simulink library "lib_controller"  (R2015a)
settings: Solver=ode45  StartTime=0.0  StopTime=10.0  RelTol=1e-3
values from neighbouring files (symbols this model uses):
  CG_0 = [0,0,0.02]'    [SetupComplete.m]
  g = 9.81    [SetupComplete.m]
  h_M = 0.064    [SetupComplete.m]
  I_BAC_0 = [ Ix,0,Ixz;0,Iy,0;Ixz,0,Iz]    [SetupComplete.m]
  l = 0.3450    (= 0.345)    [NDI_components.m]    (also in SetupComplete.m; robust_controller.m)
  m = 3.51    [SetupComplete.m]
  m_0 = 2.61    [SetupComplete.m]
  m_M = 0.300    (= 0.3)    [SetupComplete.m]
  T_sim = 0.01    [Run3Copter.m]
undefined symbols (not defined in the file or in its folder): Theta_1_roll_last, Theta_2_roll_last, Theta_3_roll_last, V_long_lastA_w_z, V_long_lastAoA, V_roll_last, V_yaw_last, W_long_lastA_w_z, W_long_lastAoA, W_roll_last, W_yaw_last
libraries: simulink x65, Adaptive_FaultTolerantControl x8, lib_controller x5, qcatlib x4, dspinverses x4, aerolibtransform2 x3, aerolib6dofsys x1
(part 2 of 10)

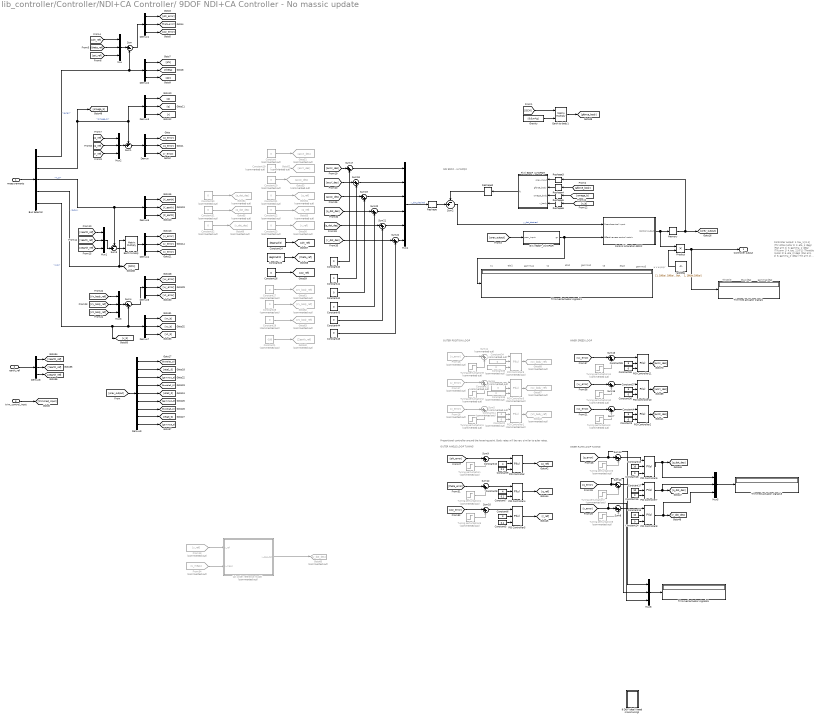
== system lib_controller/Controller/NDI+CA Controller/ 9DOF NDI+CA Controller - No massic update ==
  note: gamma3
  note: gamma2
  note: gamma1
  note: eta3
  note: eta2
  note: eta1
  note: t3
  note: t2
  note: t1
  note: u
      | v
      | w
      | p
      | q
      | r
  note: OUTER POSITION LOOP
  note: gamma[deg]
  note: eta [deg]
  note: Throttle
  note: Controller output:
      | 1. tau_1 [0-1] (Thr ottle motor 1)
      | 2. eta_1 (deg)  (Pan arm 1)
      | 3. gamma_1 (deg)  (Tilt arm 1)
      |
      | 4. tau_2 [0-1] (Throttle motor 2)
      | 5. eta_2 (deg)  (Pan arm 2)
      | 6. gamma_2 (deg)  (Tilt arm 2)
      |
      | 7. tau_3 [0-1] (Throttle motor 3)
      | 8. eta_3 (deg)  (Pan arm  3)
      | 9. gamma_3 (deg)  (Tilt arm 3)
  note: Proportional controller around the hovering point. Body rates will be very similar to euler rates.
  note: INNER RATE LOOP TUNING
  note: OUTER ANGLE LOOP TUNING
  note: INNER SPEED LOOP
  note: NDI 9DOF - UVWPQR
  measurements : Inport
  earth_ref : Inport  Port=2
  trim_control_input : Inport  Port=3
  1st order reference model : Subsystem  Commented=on  mask(1st order model reference block){Kref=1, Kb=20, fi=0.25, fc=0.5, Kf=1}
      mask prompts: Kref "1st order reference gain"; Kb "Bandwidth gain"; fi "Integral gain"; fc "Command FF gain"; Kf "Command_dot FF gain"
      mask help:
      | Generates a desired first order derivative of a commanded output taking
      | into account the current measured output.
      | Kref is the gain that determines the first order system between y_ref and
      | y_commanded signals. Ycom/Yref = Kref/(1 + Kref)
      | fi and fc can be defaulted to 0.25 and 0.5 for a critically damped 2nd
      | order response between y_meas and the error signal (y_com - y_meas) considering
      | a perfect dynamic inversion.
      mask Help:
      | Juan Herrero Macias <jn.herrerom@gmail.com>
      | This architecture can be found and explained in Fault-tolerant Flight
      | Control and Guidance Systems, Ducard, Guillaume.
      mask TypeOptions Kref: Kref gain/Gain
      mask TypeOptions Kb: Bandwidth gain/Gain
      mask TypeOptions fi: Integral gain/Gain
      mask TypeOptions fc: Command FF gain/Gain
      mask TypeOptions Kf: Command_dot FF gain/Gain
  9 DOF Ideal (Need more tuning) : Subsystem
  Bus Selector : BusSelector  OutputSignals=euler,omega_b,X_e,DCM,V_b
  Constant{,2,11..12,19..23,27..35} (18 alike) : Constant  Commented=on  Value=0
  Constant1 : Constant  Commented=on  Value=-100
  Constant10 : Constant  Value=4
  Constant13 : Constant  Value=10
  Constant{3,14,16,18,26,36,38,40..45} (13 alike) : Constant  Value=0
  Constant15 : Constant  Value=10
  Constant17 : Constant  Value=10
  Constant24 : Constant  Value=deg2rad(0)
  Constant25 : Constant  Value=deg2rad(0)
  Constant37 : Constant  Value=5
  Constant39 : Constant  Value=5
  Constant4 : Constant  Value=5
  Constant5 : Constant  Value=0.1
  Constant6 : Constant  Value=3
  Constant7 : Constant  Value=0.1
  Constant8 : Constant  Value=4
  Constant9 : Constant  Value=0.1
  Control Allocation 9DOF : Subsystem  Variant=on  OverrideUsingVariant=(default)
  Demux{,1..8} (9 alike) : Demux  Outputs=3
  Demux9 : Demux  Outputs=9
  Earth to body : Product  Multiplication=Matrix(*)
  Earth to body1 : Product  Multiplication=Matrix(*)
  F(X) 9DOF_UVWPQR : MATLAB Function  TreatAsAtomicUnit=on
  From13 : From  Commented=on  GotoTag=y_ref
  From16 : From  Commented=on  GotoTag=z_error
  From17 : From  Commented=on  GotoTag=y_error
  From18 : From  Commented=on  GotoTag=x_error
  From34 : From  Commented=on  GotoTag=y_meas
  G(X) 9DOF_UVWPQR : MATLAB Function  TreatAsAtomicUnit=on
  Goto40 : Goto  Commented=on  GotoTag=Zearth_ref
  Goto43 : Goto  Commented=on  GotoTag=Vz_body_ref
  Goto51 : Goto  Commented=on  GotoTag=accX_des
  Goto52 : Goto  Commented=on  GotoTag=accY_des
  Goto53 : Goto  Commented=on  GotoTag=accZ_des
  Goto54 : Goto  Commented=on  GotoTag=p_ref
  Goto55 : Goto  Commented=on  GotoTag=q_ref
  Goto56 : Goto  Commented=on  GotoTag=r_ref
  Goto60 : Goto  Commented=on  GotoTag=y_dot_des
  Goto61 : Goto  Commented=on  GotoTag=Vx_body_ref
  Goto62 : Goto  Commented=on  GotoTag=Vy_body_ref
  Goto63 : Goto  Commented=on  GotoTag=Vz_body_ref
  Goto64 : Goto  Commented=on  GotoTag=p_dot_des
  Goto65 : Goto  Commented=on  GotoTag=q_dot_des
  Goto66 : Goto  Commented=on  GotoTag=r_dot_des
  Goto67 : Goto  Commented=on  GotoTag=Vy_body_ref
  Goto68 : Goto  Commented=on  GotoTag=Vx_body_ref
  Gravity : Constant  Value=[0;0;m*g]
  Memory : Memory  X0=[0,0,0,0,0,0,0,0,0]  LinearizeAsDelay=on
  Mux{,1..3,5,8} (6 alike) : Mux  Inputs=3
  Mux4 : Mux  Inputs=6
  PID Controller{,2,4..8,10..11} (9 alike) : simulink/Continuous/PID Controller  Controller=PI  TimeDomain=Continuous-time  SampleTime=-1  IntegratorMethod=Forward Euler  FilterMethod=Forward Euler  Form=Parallel  UseFilter=on  ControllerParametersSource=external  P=1  I=1  D=0  N=100  InitialConditionSource=internal  InitialConditionForIntegrator=0  InitialConditionForFilter=0  ExternalReset=none  LimitOutput=off  UpperSaturationLimit=inf  LowerSaturationLimit=-inf  LinearizeAsGain=on  AntiWindupMode=none  Kb=1  TrackingMode=off  Kt=1  PParamMin=[]  PParamMax=[]  IParamMin=[]  IParamMax=[]  DParamMin=[]  DParamMax=[]  NParamMin=[]  NParamMax=[]  KbParamMin=[]  KbParamMax=[]  KtParamMin=[]  KtParamMax=[]  POutMin=[]  POutMax=[]  IOutMin=[]  IOutMax=[]  DOutMin=[]  DOutMax=[]  NOutMin=[]  NOutMax=[]  KbOutMin=[]  KbOutMax=[]  KtOutMin=[]  KtOutMax=[]  IntegratorOutMin=[]  IntegratorOutMax=[]  FilterOutMin=[]  FilterOutMax=[]  SumOutMin=[]  SumOutMax=[]  SumI1OutMin=[]  SumI1OutMax=[]  SumI2OutMin=[]  SumI2OutMax=[]  SumI3OutMin=[]  SumI3OutMax=[]  SumDOutMin=[]  SumDOutMax=[]  SaturationOutMin=[]  SaturationOutMax=[]  IntegratorContinuousStateAttributes=''  IntegratorStateMustResolveToSignalObject=off  IntegratorRTWStateStorageClass=Auto  FilterContinuousStateAttributes=''  FilterStateMustResolveToSignalObject=off  FilterRTWStateStorageClass=Auto  DifferentiatorICPrevScaledInput=0  DifferentiatorOutMin=[]  DifferentiatorOutMax=[]
  PID Controller1 : simulink/Continuous/PID Controller  Commented=on  Controller=PI  TimeDomain=Continuous-time  SampleTime=-1  IntegratorMethod=Forward Euler  FilterMethod=Forward Euler  Form=Parallel  UseFilter=on  ControllerParametersSource=external  P=1  I=1  D=0  N=100  InitialConditionSource=internal  InitialConditionForIntegrator=0  InitialConditionForFilter=0  ExternalReset=none  LimitOutput=off  UpperSaturationLimit=inf  LowerSaturationLimit=-inf  LinearizeAsGain=on  AntiWindupMode=none  Kb=1  TrackingMode=off  Kt=1  PParamMin=[]  PParamMax=[]  IParamMin=[]  IParamMax=[]  DParamMin=[]  DParamMax=[]  NParamMin=[]  NParamMax=[]  KbParamMin=[]  KbParamMax=[]  KtParamMin=[]  KtParamMax=[]  POutMin=[]  POutMax=[]  IOutMin=[]  IOutMax=[]  DOutMin=[]  DOutMax=[]  NOutMin=[]  NOutMax=[]  KbOutMin=[]  KbOutMax=[]  KtOutMin=[]  KtOutMax=[]  IntegratorOutMin=[]  IntegratorOutMax=[]  FilterOutMin=[]  FilterOutMax=[]  SumOutMin=[]  SumOutMax=[]  SumI1OutMin=[]  SumI1OutMax=[]  SumI2OutMin=[]  SumI2OutMax=[]  SumI3OutMin=[]  SumI3OutMax=[]  SumDOutMin=[]  SumDOutMax=[]  SaturationOutMin=[]  SaturationOutMax=[]  IntegratorContinuousStateAttributes=''  IntegratorStateMustResolveToSignalObject=off  IntegratorRTWStateStorageClass=Auto  FilterContinuousStateAttributes=''  FilterStateMustResolveToSignalObject=off  FilterRTWStateStorageClass=Auto  DifferentiatorICPrevScaledInput=0  DifferentiatorOutMin=[]  DifferentiatorOutMax=[]
  PID Controller3 : simulink/Continuous/PID Controller  Commented=on  Controller=PI  TimeDomain=Continuous-time  SampleTime=-1  IntegratorMethod=Forward Euler  FilterMethod=Forward Euler  Form=Parallel  UseFilter=on  ControllerParametersSource=external  P=1  I=1  D=0  N=100  InitialConditionSource=internal  InitialConditionForIntegrator=0  InitialConditionForFilter=0  ExternalReset=none  LimitOutput=off  UpperSaturationLimit=inf  LowerSaturationLimit=-inf  LinearizeAsGain=on  AntiWindupMode=none  Kb=1  TrackingMode=off  Kt=1  PParamMin=[]  PParamMax=[]  IParamMin=[]  IParamMax=[]  DParamMin=[]  DParamMax=[]  NParamMin=[]  NParamMax=[]  KbParamMin=[]  KbParamMax=[]  KtParamMin=[]  KtParamMax=[]  POutMin=[]  POutMax=[]  IOutMin=[]  IOutMax=[]  DOutMin=[]  DOutMax=[]  NOutMin=[]  NOutMax=[]  KbOutMin=[]  KbOutMax=[]  KtOutMin=[]  KtOutMax=[]  IntegratorOutMin=[]  IntegratorOutMax=[]  FilterOutMin=[]  FilterOutMax=[]  SumOutMin=[]  SumOutMax=[]  SumI1OutMin=[]  SumI1OutMax=[]  SumI2OutMin=[]  SumI2OutMax=[]  SumI3OutMin=[]  SumI3OutMax=[]  SumDOutMin=[]  SumDOutMax=[]  SaturationOutMin=[]  SaturationOutMax=[]  IntegratorContinuousStateAttributes=''  IntegratorStateMustResolveToSignalObject=off  IntegratorRTWStateStorageClass=Auto  FilterContinuousStateAttributes=''  FilterStateMustResolveToSignalObject=off  FilterRTWStateStorageClass=Auto  DifferentiatorICPrevScaledInput=0  DifferentiatorOutMin=[]  DifferentiatorOutMax=[]
  PID Controller9 : simulink/Continuous/PID Controller  Commented=on  Controller=PI  TimeDomain=Continuous-time  SampleTime=-1  IntegratorMethod=Forward Euler  FilterMethod=Forward Euler  Form=Parallel  UseFilter=on  ControllerParametersSource=external  P=1  I=1  D=0  N=100  InitialConditionSource=internal  InitialConditionForIntegrator=0  InitialConditionForFilter=0  ExternalReset=none  LimitOutput=off  UpperSaturationLimit=inf  LowerSaturationLimit=-inf  LinearizeAsGain=on  AntiWindupMode=none  Kb=1  TrackingMode=off  Kt=1  PParamMin=[]  PParamMax=[]  IParamMin=[]  IParamMax=[]  DParamMin=[]  DParamMax=[]  NParamMin=[]  NParamMax=[]  KbParamMin=[]  KbParamMax=[]  KtParamMin=[]  KtParamMax=[]  POutMin=[]  POutMax=[]  IOutMin=[]  IOutMax=[]  DOutMin=[]  DOutMax=[]  NOutMin=[]  NOutMax=[]  KbOutMin=[]  KbOutMax=[]  KtOutMin=[]  KtOutMax=[]  IntegratorOutMin=[]  IntegratorOutMax=[]  FilterOutMin=[]  FilterOutMax=[]  SumOutMin=[]  SumOutMax=[]  SumI1OutMin=[]  SumI1OutMax=[]  SumI2OutMin=[]  SumI2OutMax=[]  SumI3OutMin=[]  SumI3OutMax=[]  SumDOutMin=[]  SumDOutMax=[]  SaturationOutMin=[]  SaturationOutMax=[]  IntegratorContinuousStateAttributes=''  IntegratorStateMustResolveToSignalObject=off  IntegratorRTWStateStorageClass=Auto  FilterContinuousStateAttributes=''  FilterStateMustResolveToSignalObject=off  FilterRTWStateStorageClass=Auto  DifferentiatorICPrevScaledInput=0  DifferentiatorOutMin=[]  DifferentiatorOutMax=[]
  Product : Product
  Reshape : Reshape  OutputDimensionality=Column vector (2-D)
  Reshape2 : Reshape  OutputDimensionality=Column vector (2-D)  OutputDimensions=[6,1]
  Reshape{3..6} (4 alike) : Reshape  OutputDimensions=[6,1]
  Sum : Sum  Inputs=|+-
  Sum1 : Sum  Inputs=-+|
  Sum{7..10,12..22} (15 alike) : Sum  Inputs=|++
  Sum11 : Sum  Commented=on  Inputs=|++
  Sum2 : Sum  Inputs=-+|
  Sum3 : Sum  Inputs=-+|
  Sum4 : Sum  Inputs=|+-
  Sum5 : Sum  Commented=on  Inputs=|++
  Sum6 : Sum  Commented=on  Inputs=|++
  Trimmed actuator signals{,1,3,5} (4 alike) : Display
  Tuning perturbation{,5..6,8} (4 alike) : Step  Commented=on  Time=20  After=3*pi/180  SampleTime=0
  Tuning perturbation{1..3,9..11} (6 alike) : Step  Commented=on  Time=20  SampleTime=0
  Tuning perturbation4 : Step  Commented=on  Time=20  After=-3*pi/180  SampleTime=0
  Tuning perturbation7 : Step  Commented=on  Time=20  After=-3*pi/180  SampleTime=0
  rad2deg : Constant  Value="[1, 180/pi, 180/pi,    1,180/pi, 180/pi,     1, 180/pi,180/pi]"
  Controller output : Outport
  wires:
  PID Controller9/1 -> Goto68/1
  Tuning perturbation9/1 -> Sum11/2
  From18/1 -> Sum11/1
  Sum11/1 -> PID Controller9/1
  Constant35/1 -> PID Controller9/3
  Constant34/1 -> PID Controller9/2
  PID Controller3/1 -> Goto67/1
  Tuning perturbation2/1 -> Sum6/2
  From17/1 -> Sum6/1
  Sum6/1 -> PID Controller3/1
  Constant33/1 -> PID Controller3/3
  Constant12/1 -> PID Controller3/2
  PID Controller1/1 -> Goto43/1
  Tuning perturbation1/1 -> Sum5/2
  Sum5/1 -> PID Controller1/1
  Constant2/1 -> PID Controller1/3
  Constant11/1 -> PID Controller1/2
  Constant1/1 -> Goto40/1
  G(X) 9DOF_UVWPQR/1(gx) -> Trimmed actuator signals1/1, Control Allocation 9DOF/2(Effectiveness control matrix)
  [prev_output] -> G(X) 9DOF_UVWPQR/1(prev_input)
  Control Allocation 9DOF/1(Control output) -> Memory/1, Product/1
  Sum2/1 -> Control Allocation 9DOF/1(Pseudocontrol input)  "y_dot_desired"
  Constant13/1 -> PID Controller6/2
  Sum3/1 -> Earth to body/2
  Constant32/1 -> Goto66/1
  Constant31/1 -> Goto65/1
  Constant30/1 -> Goto64/1
  Memory/1 -> [prev_output], Reshape3/1
  [DCM] -> Earth to body1/1
  Mux8/1 -> Trimmed actuator signals5/1
  [r_error] -> Sum8/1, Mux8/3
  [q_error] -> Sum13/1, Mux8/2
  [p_error] -> Sum14/1, Mux8/1
  [psi_error] -> Sum10/1
  [theta_error] -> Sum12/1
  [phi_error] -> Sum9/1
  Constant29/1 -> Goto63/1
  Constant28/1 -> Goto62/1
  Constant27/1 -> Goto61/1
  PID Controller2/1 -> [accZ_des]
  Mux5/1 -> Trimmed actuator signals3/1
  1st order reference model/1(y_des_dot) -> Goto60/1
  From34/1 -> 1st order reference model/2(y_meas)
  From13/1 -> 1st order reference model/1(y_ref)
  rad2deg/1 -> Product/2
  Product/1 -> Controller output/1, Trimmed actuator signals/1
  Constant18/1 -> PID Controller6/3
  Constant26/1 -> [psi_ref]
  Constant25/1 -> [theta_ref]
  Constant24/1 -> [phi_ref]
  Constant23/1 -> Goto56/1
  Constant22/1 -> Goto55/1
  Constant21/1 -> Goto54/1
  Constant20/1 -> Goto53/1
  Constant19/1 -> Goto52/1
  Constant/1 -> Goto51/1
  [v_b] -> Reshape6/1
  Reshape6/1 -> F(X) 9DOF_UVWPQR/4(v_body)
  Reshape5/1 -> F(X) 9DOF_UVWPQR/3(omega_body)
  Reshape4/1 -> F(X) 9DOF_UVWPQR/2(gforce_body)
  [omega_b] -> Reshape5/1
  Reshape3/1 -> F(X) 9DOF_UVWPQR/1(prev_input)
  Reshape2/1 -> Sum2/1
  Reshape/1 -> Sum2/2
  Mux4/1 -> Reshape/1  "y_dot_desired"
  Tuning perturbation7/1 -> Sum13/2
  Tuning perturbation6/1 -> Sum14/2
  Tuning perturbation8/1 -> Sum8/2
  Sum13/1 -> PID Controller7/1
  Sum8/1 -> PID Controller8/1
  Sum14/1 -> PID Controller6/1
  Constant16/1 -> PID Controller7/3
  Constant17/1 -> PID Controller7/2
  Constant14/1 -> PID Controller8/3
  Constant15/1 -> PID Controller8/2
  PID Controller8/1 -> [r_dot_des], Mux5/3
  PID Controller7/1 -> [q_dot_des], Mux5/2
  PID Controller6/1 -> [p_dot_des], Mux5/1
  Tuning perturbation4/1 -> Sum12/2
  Tuning perturbation/1 -> Sum9/2
  Tuning perturbation5/1 -> Sum10/2
  Sum12/1 -> PID Controller4/1
  Sum10/1 -> PID Controller5/1
  Sum9/1 -> PID Controller/1
  Constant7/1 -> PID Controller4/3
  Constant9/1 -> PID Controller/3
  Constant10/1 -> PID Controller/2
  Constant8/1 -> PID Controller4/2
  Constant5/1 -> PID Controller5/3
  Constant6/1 -> PID Controller5/2
  PID Controller5/1 -> [r_ref]
  PID Controller4/1 -> [q_ref]
  PID Controller/1 -> [p_ref]
  Tuning perturbation3/1 -> Sum7/2
  [vz_error] -> Sum7/1
  Sum7/1 -> PID Controller2/1
  Constant3/1 -> PID Controller2/3
  Constant4/1 -> PID Controller2/2
  [gforce_body] -> Reshape4/1
  Earth to body1/1 -> [gforce_body]
  Gravity/1 -> Earth to body1/2
  F(X) 9DOF_UVWPQR/1(fx) -> Reshape2/1
  Mux/1 -> Sum/1
  Demux3/3 -> [r]
  Demux3/2 -> [q]
  Demux3/1 -> [p]
  Demux2/1 -> [phi]
  Demux2/2 -> [theta]
  Demux2/3 -> [psi]
  measurements/1 -> Bus Selector/1
  Bus Selector/1 -> Demux2/1, Sum/2  "<euler>"
  Bus Selector/2 -> Demux3/1, Sum1/1, [omega_b]  "<omega_b>"
  Sum1/1 -> Demux/1
  Sum/1 -> Demux1/1
  Demux/3 -> [r_error]
  Demux/2 -> [q_error]
  Demux/1 -> [p_error]
  Demux1/1 -> [phi_error]
  Demux1/2 -> [theta_error]
  Demux1/3 -> [psi_error]
  trim_control_input/1 -> [trimmed_input]
  [theta_ref] -> Mux/2
  [phi_ref] -> Mux/1
  [psi_ref] -> Mux/3
  Mux2/1 -> Sum1/2
  [q_ref] -> Mux2/2
  [p_ref] -> Mux2/1
  [r_ref] -> Mux2/3
  Bus Selector/3 -> Demux5/1, Sum3/1  "<X_e>"
  Demux5/3 -> [Z_earth]
  Demux5/2 -> [Y_earth]
  Demux5/1 -> [X_earth]
  Demux4/3 -> [z_error]
  Demux4/2 -> [y_error]
  Demux4/1 -> [x_error]
  Mux1/1 -> Sum3/2
  [Yearth_ref] -> Mux1/2
  [Xearth_ref] -> Mux1/1
  [Zearth_ref] -> Mux1/3
  Mux3/1 -> Sum4/1
  Demux7/1 -> [vx_b]
  Demux7/2 -> [vy_b]
  Demux7/3 -> [vz_b]
  Bus Selector/5 -> Demux7/1, Sum4/2, [v_b]  "<V_b>"
  Sum4/1 -> Demux6/1
  Demux6/1 -> [vx_error]
  Demux6/2 -> [vy_error]
  Demux6/3 -> [vz_error]
  [Vy_body_ref] -> Mux3/2
  [Vx_body_ref] -> Mux3/1
  [Vz_body_ref] -> Mux3/3
  Bus Selector/4 -> [DCM], Earth to body/1  "<DCM>"
  Earth to body/1 -> Demux4/1
  Demux8/3 -> [Zearth_ref]
  Demux8/2 -> [Yearth_ref]
  Demux8/1 -> [Xearth_ref]
  earth_ref/1 -> Demux8/1
  [prev_output] -> Demux9/1
  Demux9/1 -> [throttle1_0]
  Demux9/2 -> [eta1_0]
  Demux9/3 -> [gamma1_0]
  Demux9/4 -> [throttle2_0]
  Demux9/5 -> [eta2_0]
  Demux9/6 -> [gamma2_0]
  Demux9/7 -> [throttle3_0]
  Demux9/8 -> [eta3_0]
  Demux9/9 -> [gamma3_0]
  PID Controller10/1 -> [accY_des]
  Tuning perturbation10/1 -> Sum15/2
  [vy_error] -> Sum15/1
  Sum15/1 -> PID Controller10/1
  Constant36/1 -> PID Controller10/3
  Constant37/1 -> PID Controller10/2
  PID Controller11/1 -> [accX_des]
  Tuning perturbation11/1 -> Sum16/2
  [vx_error] -> Sum16/1
  Sum16/1 -> PID Controller11/1
  Constant38/1 -> PID Controller11/3
  Constant39/1 -> PID Controller11/2
  From16/1 -> Sum5/1
  [accX_des] -> Sum17/1
  [accY_des] -> Sum18/1
  [accZ_des] -> Sum19/1
  [p_dot_des] -> Sum20/1
  [q_dot_des] -> Sum21/1
  [r_dot_des] -> Sum22/1
  Constant40/1 -> Sum17/2
  Constant41/1 -> Sum18/2
  Constant42/1 -> Sum19/2
  Constant43/1 -> Sum20/2
  Constant44/1 -> Sum21/2
  Constant45/1 -> Sum22/2
  Sum22/1 -> Mux4/6
  Sum21/1 -> Mux4/5
  Sum20/1 -> Mux4/4
  Sum19/1 -> Mux4/3
  Sum18/1 -> Mux4/2
  Sum17/1 -> Mux4/1

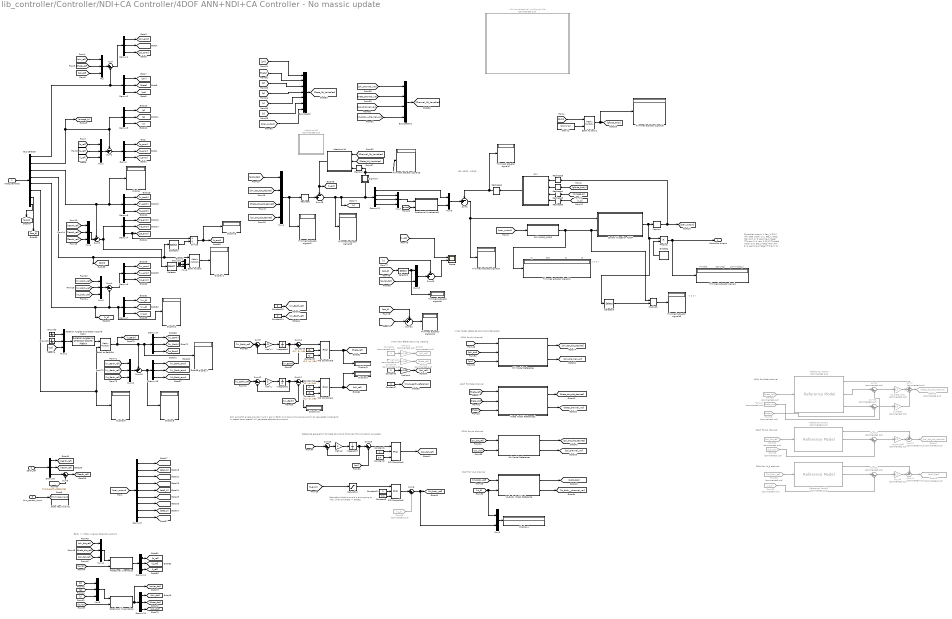
== system lib_controller/Controller/NDI+CA Controller/4DOF ANN+NDI+CA Controller - No massic update ==
  note: Roll and pitch angle provide X and Y acc in Earth axis (around hovering point). So requested increments in speed (error speed) will generate attitude commands
  note: Saturation block to avoid z_error going to
      |  infty when phi/theta -> 90deg
  note: Inner loop reference tuning / testing
  note: Earth <-> Body Angular Rate Conversions
  note: Reference generation for Rate Command Channels (for simulation purposes)
  note: ACAH for phi channel
  note: NDI 4DOF - WPQR
  note: Controller output:
      | 1. tau_1 [0-1] (Thr ottle motor 1)
      | 2. eta_1 (deg)  (Pan arm 1)
      | 3. gamma_1 (deg)  (Tilt arm 1)
      |
      | 4. tau_2 [0-1] (Throttle motor 2)
      | 5. eta_2 (deg)  (Pan arm 2)
      | 6. gamma_2 (deg)  (Tilt arm 2)
      |
      | 7. tau_3 [0-1] (Throttle motor 3)
      | 8. eta_3 (deg)  (Pan arm  3)
      | 9. gamma_3 (deg)  (Tilt arm 3)
  note: Throttle
  note: eta [deg]
  note: gamma[deg]
  note: eta1
  note: t3
  note: t2
  note: t1
  note: w
      | p
      | q
      | r
  note: ACAH for theta channel
  note: RCAH for psi channel
  note: RCAH for Vz_b channel
  note: Inner Model reference Command Generator
  note: ACAH for theta channel
  note: RCAH for psi channel
  note: RCAH for Vz_b channel
  note: w
      | p
      | q
      | r
  measurements : Inport
  earth_ref : Inport  Port=2
  trim_control_input : Inport  Port=3
  Adaptive NN : Subsystem  Variant=on  VariantControl=Variant  OverrideUsingVariant=NN on AoA
      mask Display:
      | image(imread('ANN.png'))
      | 
      | 
      | port_label('input', 2, 'State vars')
      | port_label('input', 1, 'Channel vars')
      | port_label('input', 3, 'v prev')
      | 
      | port_label('output', 1, 'v_ad^')
  Adaptive NN1 : Subsystem  Commented=on  Variant=on  VariantControl=Variant  OverrideUsingVariant=NN on AoA
      mask Display:
      | image(imread('ANN.png'))
      | 
      | 
      | port_label('input', 2, 'State vars')
      | port_label('input', 1, 'Channel vars')
      | port_label('input', 3, 'v prev')
      | 
      | port_label('output', 1, 'v_ad^')
  Bus Creator : BusCreator  Inputs=7
  Bus Creator1 : BusCreator
  Bus Selector : BusSelector  OutputSignals=euler,omega_b,X_e,DCM,V_b,V_e,A_b,A_s
  Constant1 : Constant  Value=4
  Constant10 : Constant  Value=10 * pi /180
  Constant11 : Constant
  Constant12 : Constant  Value=0.2 * pi /180
  Constant13 : Constant  Value=5
  Constant14 : Constant  Value=0
  Constant2 : Constant  Value=0.4
  Constant3 : Constant  Value=0.1
  Constant4 : Constant  Commented=on  Value=0
  Constant5 : Constant  Commented=on  Value=0
  Constant6 : Constant  Value=0
  Constant7 : Constant  Value=0
  Constant8 : Constant  Value=-10 * pi /180
  Constant9 : Constant  Value=-0.2 * pi /180
  Control Allocation 4DOF : Subsystem  Variant=on  OverrideUsingVariant=Variant1
  Demux{,1..8,10..11,13..14} (13 alike) : Demux  Outputs=3
  Demux12 : Demux
  Demux9 : Demux  Outputs=9
  Display{,1..10} (11 alike) : Display
  Divide : Product  Inputs=*/
  Earth to EarthPsi : Product  Multiplication=Matrix(*)
  Earth to body : Product  Multiplication=Matrix(*)
  Earth to body1 : Product  Multiplication=Matrix(*)
  F(X) : MATLAB Function  TreatAsAtomicUnit=on
  From29 : From  Commented=on  GotoTag=theta
  From33 : From  Commented=on  GotoTag=psi_dot_ref
  From36 : From  Commented=on  GotoTag=Vz_body_ref
  From38 : From  Commented=on  GotoTag=theta_ref
  From39 : From  Commented=on  GotoTag=vz_b
  From47 : From  Commented=on  GotoTag=theta_dot
  From49 : From  Commented=on  GotoTag=psi_dot
  From65 : From  Commented=on  GotoTag=vz_b
  G(X) 4DOF_WPQR : MATLAB Function  TreatAsAtomicUnit=on
  Goto Tag Visibility : GotoTagVisibility  GotoTag=trimmed_input
  Goto45 : Goto  Commented=on  GotoTag=theta_dot_dot_desired
  Goto47 : Goto  Commented=on  GotoTag=psi_dot_dot_desired
  Goto48 : Goto  Commented=on  GotoTag=accZ_des
  Goto57 : Goto  Commented=on  GotoTag=phi_ref
  Goto58 : Goto  Commented=on  GotoTag=theta_ref
  Gravity : Constant  Value=[0;0;m*g]
  Ground{,1..3} (4 alike) : Ground
  Integrator1 : Integrator
  Integrator2 : Integrator
  Integrator7 : Integrator
  Ki_theta1 : Gain  Commented=on  Gain=0.5
  Kp_psi_dot1 : Gain  Commented=on  Gain=0.5
  Kp_theta_dot1 : Gain  Commented=on  Gain=0.5
  Kp_vz1 : Gain  Commented=on  Gain=0.5
  Kref psi : Gain
  Kref psi1 : Gain  Commented=on  Gain=pi/180
  Kref psi2 : Gain  Commented=on  Gain=pi/180
  Kref psi4 : Gain  Gain=pi/180
  Kref vx : Gain  Gain=-5
  Kref vy : Gain  Gain=5
  Memory : Memory  X0=[0,0,0,0,0,0,0,0,0]  LinearizeAsDelay=on
  Memory1 : Memory
  Mux{,1..3,5..7,10..12} (10 alike) : Mux  Inputs=3
  Mux13 : Mux  Inputs=2
  Mux4 : Mux
  Mux8 : Mux  Inputs=2
  Mux9 : Mux  Inputs=2
  On-line (adaptive) multi-layer NNs : Subsystem  Commented=on
      mask Display:
      | image(imread('ANN.png'))
      | 
      | port_label('input', 1, 'v prev')
      | port_label('input', 2, 'All meas')
      | port_label('input', 3, 'NN vars')
      | 
      | port_label('output', 1, 'v_ad^')
  PID Controller{1..4} (4 alike) : simulink/Continuous/PID Controller  Controller=PI  TimeDomain=Continuous-time  SampleTime=-1  IntegratorMethod=Forward Euler  FilterMethod=Forward Euler  Form=Parallel  UseFilter=on  ControllerParametersSource=external  P=1  I=1  D=0  N=100  InitialConditionSource=internal  InitialConditionForIntegrator=0  InitialConditionForFilter=0  ExternalReset=none  LimitOutput=off  UpperSaturationLimit=inf  LowerSaturationLimit=-inf  LinearizeAsGain=on  AntiWindupMode=none  Kb=1  TrackingMode=off  Kt=1  PParamMin=[]  PParamMax=[]  IParamMin=[]  IParamMax=[]  DParamMin=[]  DParamMax=[]  NParamMin=[]  NParamMax=[]  KbParamMin=[]  KbParamMax=[]  KtParamMin=[]  KtParamMax=[]  POutMin=[]  POutMax=[]  IOutMin=[]  IOutMax=[]  DOutMin=[]  DOutMax=[]  NOutMin=[]  NOutMax=[]  KbOutMin=[]  KbOutMax=[]  KtOutMin=[]  KtOutMax=[]  IntegratorOutMin=[]  IntegratorOutMax=[]  FilterOutMin=[]  FilterOutMax=[]  SumOutMin=[]  SumOutMax=[]  SumI1OutMin=[]  SumI1OutMax=[]  SumI2OutMin=[]  SumI2OutMax=[]  SumI3OutMin=[]  SumI3OutMax=[]  SumDOutMin=[]  SumDOutMax=[]  SaturationOutMin=[]  SaturationOutMax=[]  IntegratorContinuousStateAttributes=''  IntegratorStateMustResolveToSignalObject=off  IntegratorRTWStateStorageClass=Auto  FilterContinuousStateAttributes=''  FilterStateMustResolveToSignalObject=off  FilterRTWStateStorageClass=Auto  DifferentiatorICPrevScaledInput=0  DifferentiatorOutMin=[]  DifferentiatorOutMax=[]
  Phi Model Reference : Subsystem  mask{omega_n=8, xi=1.1, r=1}
      mask prompts: omega_n "Natural Frequency"; xi "Damping"; r "NN Error dynamic ratio"
      mask help:
      | 2nd Order Model Reference System
      | Natural frequency and damping ratio set the dynamic of the model reference.
      | Error dynamic ratio sets how faster compared to the reference model dynamics
      | is the settling time of the inversion error provided by the NN.
      mask Display:
      | TF = tf([omega_n^2],[1 xi*omega_n omega_n^2]);
      | 
      | [y,t]=step(TF);
      | S = stepinfo(y,t);
      | 
      | pos = get_param(gcb, 'Position');
      | width = pos(3) - pos(1);
      | height = pos(4) - pos(2);
      | t = t.*width/max(t);
      | y=y.*height/max(y);
      | plot(t,y);
      | S2 = stepinfo(y,t);
      | 
      | if S.Overshoot==0 % 1st order response
      |     text(S2.RiseTime ,height*0.85,['Rise time = ',num2str(S.RiseTime),'s' ]);
      |     text(S2.RiseTime ,height*0.75,['Settling Time = ',num2str(S.SettlingTime)]);
      | 
      | elseif S.Overshoot<0.05 % 2nd order response
      |     text(width*0.5 ,height*0.9,['Rise time = ',num2str(S.RiseTime),'s' ]);
      |     text(width*0.5 ,height*0.8,['Pike time = ',num2str(S.PeakTime),'s' ]);
      |     text(width*0.5 ,height*0.7,['Os = ',num2str(S.Peak)]);
      |     text(width*0.5 ,height*0.6,['SettlingTime = ',num2str(S.SettlingTime)]);
      | else % 2nd order response
      |     text(S2.PeakTime ,S2.Peak*0.85,['Peak time = ',num2str(S.PeakTime),'s' ]);
      |     text(S2.PeakTime ,S2.Peak*0.75,['Os = ',num2str(S.Peak)]);
      |     text(S2.PeakTime ,S2.Peak*0.65,['SettlingTime = ',num2str(S.SettlingTime)]);
      | end
      | 
      | 
      | [num,den] = tfdata(TF);
      | dpoly(num{:},den{:}, 's');
  Product : Product
  Product1 : Product  Multiplication=Matrix(*)
  Psi Model Reference : Subsystem  mask{tau=0.15, r=1}
      mask prompts: tau "Time Constant"; r "NN Error dynamic ratio"
      mask help:
      | 1st Order Model Reference System
      | Tau is the time constant and sets the dynamics of the reference model.
      | Error dynamic ratio sets how faster compared to the reference model is the
      | NN output going to try to compensate for the inversion error.
      mask Display:
      | K_ref=1/tau;
      | TF = tf([K_ref],[1 K_ref]);
      | 
      | [y,t]=step(TF);
      | S = stepinfo(y,t);
      | 
      | pos = get_param(gcb, 'Position');
      | width = pos(3) - pos(1);
      | height = pos(4) - pos(2);
      | t = t.*width/max(t);
      | y=y.*height/max(y);
      | plot(t,y);
      | S2 = stepinfo(y,t);
      | 
      | if S.Overshoot==0 % 1st order response
      |     text(S2.RiseTime ,height*0.85,['Rise time = ',num2str(S.RiseTime),'s' ]);
      |     text(S2.RiseTime ,height*0.75,['Settling Time = ',num2str(S.SettlingTime)]);
      | 
      | elseif S.Overshoot<0.05 % 2nd order response
      |     text(width*0.5 ,height*0.9,['Rise time = ',num2str(S.RiseTime),'s' ]);
      |     text(width*0.5 ,height*0.8,['Pike time = ',num2str(S.PeakTime),'s' ]);
      |     text(width*0.5 ,height*0.7,['Os = ',num2str(S.Peak)]);
      |     text(width*0.5 ,height*0.6,['SettlingTime = ',num2str(S.SettlingTime)]);
      | else % 2nd order response
      |     text(S2.PeakTime ,S2.Peak*0.85,['Peak time = ',num2str(S.PeakTime),'s' ]);
      |     text(S2.PeakTime ,S2.Peak*0.75,['Os = ',num2str(S.Peak)]);
      |     text(S2.PeakTime ,S2.Peak*0.65,['SettlingTime = ',num2str(S.SettlingTime)]);
      | end
      | 
      | 
      | [num,den] = tfdata(TF);
      | dpoly(num{:},den{:}, 's');
  Reference Model1 : Adaptive_FaultTolerantControl/Ref Model and P Controller/Reference Model  Commented=on  omega_n=omega_n  xi=xi
  Reference Model4 : Adaptive_FaultTolerantControl/Ref Model and P Controller/Reference Model  Commented=on  omega_n=2.5  xi=1.1
  Reference Model5 : Adaptive_FaultTolerantControl/Ref Model and P Controller/Reference Model  Commented=on  omega_n=omega_n  xi=xi
  Reshape : Reshape
  Reshape2 : Reshape  OutputDimensionality=Column vector (2-D)  OutputDimensions=[6,1]
  Reshape{3..6} (4 alike) : Reshape  OutputDimensions=[6,1]
  Rotation Angles to Direction Cosine Matrix : aerolibtransform2/Rotation Angles to Direction Cosine Matrix  rotationOrder=ZYX
  Rotational Kinematics : MATLAB Function  TreatAsAtomicUnit=on
  Rotational Kinematics1 : MATLAB Function  TreatAsAtomicUnit=on
  Rotational Kinematics2 : MATLAB Function  TreatAsAtomicUnit=on
  Saturation : Saturate  UpperLimit=4  LowerLimit=-4
  Scope : Scope  NumInputPorts=2
      settings: ShowLegends=on  YMin=-5~-20  YMax=15~20  SaveName=ScopeData5
  Selector : Selector  InputPortWidth=3  Indices=[3]
  Selector1 : Selector  NumberOfDimensions=2  InputPortWidth=[9]  IndexOptions=Index vector (dialog),Index vector (dialog)  Indices=3,3  OutputSizes=1,1
  Selector2 : Selector  InputPortWidth=3  Indices=[3]
  Selector3 : Selector  InputPortWidth=9  Indices=[1 2 4 7]
  "Sigmoid " : Subsystem  mask{a=0.15}
      mask prompts: a "Sigmoid a param"
      mask TypeOptions a: a/Value
      mask Display:
      | x=-25:0.1:25;
      | 
      | y=(2.0 ./ (1.0 + exp(-a.*x))-1) ;
      | y2=zeros(size(x));
      | 
      | plot(x,y,x,y2);
      | 
      | %text(-20,0.5, ['a= ',num2str(a)])
  Sum{,4..5,10,12,17,25..26} (8 alike) : Sum  Inputs=|+-
  Sum{1..3,18..20} (6 alike) : Sum  Inputs=-+|
  Sum11 : Sum  Commented=on  Inputs=+-|
  Sum{8,13,15..16} (4 alike) : Sum  Commented=on  Inputs=|+-
  Sum14 : Sum  Commented=on  Inputs=+-|
  Sum21 : Sum  Inputs=++|
  Sum6 : Sum  Inputs=|++
  Sum7 : Sum  Commented=on  Inputs=+--
  Sum9 : Sum  Inputs=|++
  Theta Model Reference1 : Subsystem  mask{omega_n=8, xi=1.1, r=1}
      mask prompts: omega_n "Natural Frequency"; xi "Damping"; r "NN Error dynamic ratio"
      mask help:
      | 2nd Order Model Reference System
      | Natural frequency and damping ratio set the dynamic of the model reference.
      | Error dynamic ratio sets how faster compared to the reference model dynamics
      | is the settling time of the inversion error provided by the NN.
      mask Display:
      | TF = tf([omega_n^2],[1 xi*omega_n omega_n^2]);
      | 
      | [y,t]=step(TF);
      | S = stepinfo(y,t);
      | 
      | pos = get_param(gcb, 'Position');
      | width = pos(3) - pos(1);
      | height = pos(4) - pos(2);
      | t = t.*width/max(t);
      | y=y.*height/max(y);
      | plot(t,y);
      | S2 = stepinfo(y,t);
      | 
      | if S.Overshoot==0 % 1st order response
      |     text(S2.RiseTime ,height*0.85,['Rise time = ',num2str(S.RiseTime),'s' ]);
      |     text(S2.RiseTime ,height*0.75,['Settling Time = ',num2str(S.SettlingTime)]);
      | 
      | elseif S.Overshoot<0.05 % 2nd order response
      |     text(width*0.5 ,height*0.9,['Rise time = ',num2str(S.RiseTime),'s' ]);
      |     text(width*0.5 ,height*0.8,['Pike time = ',num2str(S.PeakTime),'s' ]);
      |     text(width*0.5 ,height*0.7,['Os = ',num2str(S.Peak)]);
      |     text(width*0.5 ,height*0.6,['SettlingTime = ',num2str(S.SettlingTime)]);
      | else % 2nd order response
      |     text(S2.PeakTime ,S2.Peak*0.85,['Peak time = ',num2str(S.PeakTime),'s' ]);
      |     text(S2.PeakTime ,S2.Peak*0.75,['Os = ',num2str(S.Peak)]);
      |     text(S2.PeakTime ,S2.Peak*0.65,['SettlingTime = ',num2str(S.SettlingTime)]);
      | end
      | 
      | 
      | [num,den] = tfdata(TF);
      | dpoly(num{:},den{:}, 's');
  Trimmed actuator signals{,1..10} (11 alike) : Display
  Vz_body Model Reference : Subsystem  mask{tau=0.3, r=1}
      mask prompts: tau "Time Constant"; r "NN Error dynamic ratio"
      mask help:
      | 1st Order Model Reference System
      | Tau is the time constant and sets the dynamics of the reference model.
      | Error dynamic ratio sets how faster compared to the reference model is the
      | NN output going to try to compensate for the inversion error.
      mask Display:
      | K_ref=1/tau;
      | TF = tf([K_ref],[1 K_ref]);
      | 
      | [y,t]=step(TF);
      | S = stepinfo(y,t);
      | 
      | pos = get_param(gcb, 'Position');
      | width = pos(3) - pos(1);
      | height = pos(4) - pos(2);
      | t = t.*width/max(t);
      | y=y.*height/max(y);
      | plot(t,y);
      | S2 = stepinfo(y,t);
      | 
      | if S.Overshoot==0 % 1st order response
      |     text(S2.RiseTime ,height*0.85,['Rise time = ',num2str(S.RiseTime),'s' ]);
      |     text(S2.RiseTime ,height*0.75,['Settling Time = ',num2str(S.SettlingTime)]);
      | 
      | elseif S.Overshoot<0.05 % 2nd order response
      |     text(width*0.5 ,height*0.9,['Rise time = ',num2str(S.RiseTime),'s' ]);
      |     text(width*0.5 ,height*0.8,['Pike time = ',num2str(S.PeakTime),'s' ]);
      |     text(width*0.5 ,height*0.7,['Os = ',num2str(S.Peak)]);
      |     text(width*0.5 ,height*0.6,['SettlingTime = ',num2str(S.SettlingTime)]);
      | else % 2nd order response
      |     text(S2.PeakTime ,S2.Peak*0.85,['Peak time = ',num2str(S.PeakTime),'s' ]);
      |     text(S2.PeakTime ,S2.Peak*0.75,['Os = ',num2str(S.Peak)]);
      |     text(S2.PeakTime ,S2.Peak*0.65,['SettlingTime = ',num2str(S.SettlingTime)]);
      | end
      | 
      | 
      | [num,den] = tfdata(TF);
      | dpoly(num{:},den{:}, 's');
  rad2deg : Constant  Value=[1, 180/pi, 0,1,0, 0, 1, 0,0]
  Controller output : Outport
  tag scope: trimmed_input=scoped
  wires:
  Demux9/9 -> [gamma3_0]
  Demux9/8 -> [eta3_0]
  Demux9/7 -> [throttle3_0]
  Demux9/6 -> [gamma2_0]
  Demux9/5 -> [eta2_0]
  Demux9/4 -> [throttle2_0]
  Demux9/3 -> [gamma1_0]
  Demux9/2 -> [eta1_0]
  Demux9/1 -> [throttle1_0]
  [prev_output] -> Demux9/1
  earth_ref/1 -> Demux8/1
  Demux8/1 -> [Xearth_ref]
  Demux8/2 -> [Yearth_ref]
  Bus Selector/4 -> Earth to body/1, Selector1/1, [DCM]  "<DCM>"
  [Vz_body_ref] -> Mux3/3
  [Vx_body_ref] -> Mux3/1
  [Vy_body_ref] -> Mux3/2
  Demux6/3 -> [vz_error]
  Demux6/2 -> [vy_error]
  Demux6/1 -> [vx_error]
  Sum4/1 -> Demux6/1
  Bus Selector/5 -> [v_b], Sum4/2, Display2/1, Demux7/1  "<V_b>"
  Demux7/3 -> [vz_b]
  Demux7/2 -> [vy_b]
  Demux7/1 -> [vx_b]
  Mux3/1 -> Sum4/1
  [Zearth_ref] -> Mux1/3
  [Xearth_ref] -> Mux1/1
  [Yearth_ref] -> Mux1/2
  Mux1/1 -> Sum3/2
  Demux4/1 -> [Xe_error]
  Demux4/2 -> [Ye_error]
  Demux4/3 -> Divide/1, [Ze_error]
  Demux5/1 -> [X_earth]
  Demux5/2 -> [Y_earth]
  Demux5/3 -> [Z_earth]
  Bus Selector/3 -> Display/1, Demux5/1, Sum3/1  "<X_e>"
  [r_ref] -> Mux2/3
  [p_ref] -> Mux2/1
  [q_ref] -> Mux2/2
  Mux2/1 -> Sum1/2
  [psi_ref] -> Mux/3
  [phi_ref] -> Mux/1
  [theta_ref] -> Mux/2
  trim_control_input/1 -> [trimmed_input]
  Demux1/3 -> [psi_error]
  Demux1/2 -> [theta_error]
  Demux1/1 -> [phi_error]
  Demux/1 -> [p_error]
  Demux/2 -> [q_error]
  Demux/3 -> [r_error]
  Sum/1 -> Demux1/1
  Sum1/1 -> Demux/1
  Bus Selector/2 -> [omega_b], Sum1/1, Demux3/1  "<omega_b>"
  Bus Selector/1 -> Sum/2, Demux2/1  "<euler>"
  measurements/1 -> Bus Selector/1
  Demux2/3 -> [psi]
  Demux2/2 -> [theta]
  Demux2/1 -> [phi]
  Demux3/1 -> [p]
  Demux3/2 -> [q]
  Demux3/3 -> [r]
  Mux/1 -> Sum/1
  F(X)/1(fx) -> Reshape2/1
  Gravity/1 -> Earth to body1/2
  Earth to body1/1 -> Trimmed actuator signals6/1, [gforce_body]
  [gforce_body] -> Reshape4/1
  Mux4/1 -> Trimmed actuator signals2/1, Reshape/1  "y_dot_desired"
  Reshape2/1 -> Sum2/1, Trimmed actuator signals7/1
  Reshape3/1 -> F(X)/1(prev_input)
  [omega_b] -> Reshape5/1
  Reshape4/1 -> F(X)/2(gforce_body)
  Reshape5/1 -> F(X)/3(omega_body)
  Reshape6/1 -> F(X)/4(v_body)
  [v_b] -> Reshape6/1
  Product/1 -> Trimmed actuator signals/1, Controller output/1
  rad2deg/1 -> Product/2
  [DCM] -> Earth to body1/1
  Memory/1 -> Reshape3/1, [prev_output]
  Sum3/1 -> Demux4/1, Selector/1
  Sum2/1 -> Trimmed actuator signals4/1, Control Allocation 4DOF/1(Pseudocontrol input)  "y_dot_desired"
  Control Allocation 4DOF/1(Control output) -> Selector3/1, Product/1, Memory/1
  [prev_output] -> G(X) 4DOF_WPQR/1(prev_input)
  [accZ_des] -> Mux4/1
  G(X) 4DOF_WPQR/1(gx) -> Trimmed actuator signals1/1, Product1/1, Control Allocation 4DOF/2(Effectiveness control matrix)
  Selector/1 -> Mux6/3
  Ground/1 -> Mux6/1
  Ground1/1 -> Mux6/2
  Mux6/1 -> Earth to body/2
  Earth to body/1 -> Display1/1
  Sum18/1 -> Trimmed actuator signals3/1, Demux12/1, "Sigmoid "/1(In), [v]  "upsilon"
  Reshape/1 -> Sum18/2  "v_o"
  Adaptive NN/1(v_ad^) -> [v_ad], Sum18/1  "v_ad"
  "Sigmoid "/1(Out) -> Trimmed actuator signals5/1, Memory1/1
  Memory1/1 -> Adaptive NN/3(v_ad^ prev)
  [euler] -> Rotational Kinematics/2(Euler)
  Demux11/1 -> [p_ref]
  Demux11/2 -> [q_ref]
  Demux11/3 -> [r_ref]
  Rotational Kinematics/1(PQR) -> Demux11/1
  [phi_dot_ref] -> Mux11/1
  [theta_dot_ref] -> Mux11/2
  [psi_dot_ref] -> Mux11/3
  Mux11/1 -> Rotational Kinematics/1(Eulerdot)
  [euler] -> Rotational Kinematics1/2(Euler)
  Mux5/1 -> Rotational Kinematics1/1(PQR)
  [r] -> Mux5/3
  [p] -> Mux5/1
  [q] -> Mux5/2
  Demux10/1 -> [phi_dot]
  Demux10/2 -> [theta_dot]
  Demux10/3 -> [psi_dot]
  Rotational Kinematics1/1(Eulerdot) -> [euler_dot], Demux10/1
  Theta Model Reference1/1(y_dot_dot_des) -> [theta_dot_dot_desired]
  [phi_dot_dot_desired] -> Mux4/2
  [theta_dot_dot_desired] -> Mux4/3
  [psi_dot_dot_desired] -> Mux4/4
  Demux12/2 -> Mux7/1  "v_phi"
  Demux12/3 -> Mux7/2  "v_theta"
  Demux12/4 -> Mux7/3  "v_psi"
  Mux7/1 -> Rotational Kinematics2/1(Eulerdot)
  [euler] -> Rotational Kinematics2/2(Euler)
  Mux8/1 -> Sum2/2  "upsilon_b"
  Demux12/1 -> Mux8/1  "v_z"
  Rotational Kinematics2/1(PQR) -> Mux8/2  "upsilon_body"
  Integrator7/1 -> Sum26/1, Sum25/2  "psi_c"
  Kref psi/1 -> Integrator7/1
  Sum25/1 -> Kref psi/1
  [psi_ref] -> Sum25/1
  [psi] -> Sum26/2
  PID Controller1/1 -> [psi_dot_ref]  "psi_dot_ref"
  Constant1/1 -> PID Controller1/2
  Constant2/1 -> PID Controller1/3
  Sum26/1 -> PID Controller1/1  "psi_error"
  Vz_body Model Reference/1(y_dot_des) -> [accZ_des]
  [Vz_body_ref] -> Vz_body Model Reference/1(u_ref)
  Constant11/1 -> PID Controller2/2
  Constant3/1 -> PID Controller2/3
  [z_error] -> Saturation/1
  PID Controller2/1 -> Sum6/1
  Selector1/1 -> Divide/2
  Divide/1 -> Display3/1, [z_error]
  [phi_ref] -> Phi Model Reference/1(u_ref)
  [phi_dot] -> Phi Model Reference/2(y_dot)
  [phi] -> Phi Model Reference/3(y)
  Phi Model Reference/1(y_dot_dot_des) -> [phi_dot_dot_desired]
  From29/1 -> Sum16/2
  Sum16/1 -> Ki_theta1/1  "theta_error"
  From38/1 -> Reference Model4/1
  Reference Model4/2 -> Sum8/1  "theta_dot_c"
  From47/1 -> Sum8/2
  Sum8/1 -> Kp_theta_dot1/1  "theta_dot_error"
  Ki_theta1/1 -> Sum7/3
  Kp_theta_dot1/1 -> Sum7/2
  Sum7/1 -> Goto45/1
  Reference Model1/2 -> Sum13/1  "psi_dot_c"
  Reference Model1/1 -> Sum11/1  "psi_dot_dot_c"
  From49/1 -> Sum13/2
  Sum13/1 -> Kp_psi_dot1/1  "psi_dot_error"
  Kp_psi_dot1/1 -> Sum11/2
  Sum11/1 -> Goto47/1
  Reference Model4/3 -> Sum16/1  "theta_c"
  From33/1 -> Reference Model1/1
  Reference Model5/2 -> Sum15/1  "vz_b_c"
  Reference Model5/1 -> Sum14/1  "accZ_c"
  From39/1 -> Sum15/2
  Sum15/1 -> Kp_vz1/1  "vz_error"
  Kp_vz1/1 -> Sum14/2
  Sum14/1 -> Goto48/1
  From36/1 -> Reference Model5/1
  Reference Model4/1 -> Sum7/1  "theta_dot_dot"
  [theta_ref] -> Theta Model Reference1/1(u_ref)
  [theta_dot] -> Theta Model Reference1/2(y_dot)
  [theta] -> Theta Model Reference1/3(y)
  [psi_dot_ref] -> Psi Model Reference/1(u_ref)
  [psi_dot] -> Psi Model Reference/2(y_dot)
  Psi Model Reference/1(y_dot_des) -> [psi_dot_dot_desired]
  [vz_b] -> Mux9/1, Vz_body Model Reference/2(y_dot)
  Phi Model Reference/2(NN_variables) -> [phi_channel_var]
  Vz_body Model Reference/2(NN_variables) -> [Vz_body__channel_var]
  Psi Model Reference/2(NN_variables) -> [psi_channel_var]
  Theta Model Reference1/2(NN_variables) -> [theta_channel_var]
  [p] -> Bus Creator/3  "p"
  [theta] -> Bus Creator/2  "theta"
  [q] -> Bus Creator/4  "q"
  [phi] -> Bus Creator/1  "phi"
  [r] -> Bus Creator/5  "r"
  Bus Creator/1 -> [State_NN_Variables]
  [State_NN_Variables] -> Adaptive NN/2(System State Vars)
  [Vz_body__channel_var] -> Bus Creator1/4  "vertical acc channel"
  [psi_channel_var] -> Bus Creator1/3  "yaw channel"
  [theta_channel_var] -> Bus Creator1/2  "pitch channel"
  [phi_channel_var] -> Bus Creator1/1  "roll channel"
  Bus Creator1/1 -> [Channel_NN_Variables]
  [Channel_NN_Variables] -> Adaptive NN/1(Model Reference Vars)
  [prev_output] -> Bus Creator/7  "prev_outputs"
  [w] -> Bus Creator/6  "w"
  Constant4/1 -> Kref psi1/1
  Constant5/1 -> Kref psi2/1
  Constant6/1 -> Kref psi4/1
  Kref psi1/1 -> Goto57/1
  Kref psi2/1 -> Goto58/1
  Kref psi4/1 -> [psi_ref]
  Mux9/1 -> Display4/1
  Demux8/3 -> Sum5/1
  Sum5/1 -> [Zearth_ref]
  Constant7/1 -> [Inc_Z_earth_reference]
  [Inc_Z_earth_reference] -> Sum5/2
  From65/1 -> Sum6/2
  Sum6/1 -> Mux9/2, [Vz_body_ref]
  Integrator1/1 -> Sum10/1, Sum9/2  "vx_c"
  Kref vx/1 -> Integrator1/1
  Sum9/1 -> Kref vx/1
  [Vx_Earth_ref] -> Sum9/1
  [Vx_Earth] -> Sum10/2
  Constant8/1 -> PID Controller3/2
  Constant9/1 -> PID Controller3/3
  Sum10/1 -> PID Controller3/1  "vx_error"
  Integrator2/1 -> Sum17/1, Sum12/2  "vy_c"
  Kref vy/1 -> Integrator2/1
  Sum12/1 -> Kref vy/1
  [Vy_Earth_ref] -> Sum12/1
  [Vy_Earth] -> Sum17/2
  Constant10/1 -> PID Controller4/2
  Constant12/1 -> PID Controller4/3
  Sum17/1 -> Display10/1, PID Controller4/1  "vy_error"
  Constant13/1 -> [Vx_Earth_ref]
  Constant14/1 -> [Vy_Earth_ref]
  Saturation/1 -> PID Controller2/1
  [Vz_Earth_ref] -> Mux10/3
  [Vx_Earth_ref] -> Mux10/1
  [Vy_Earth_ref] -> Mux10/2
  Demux13/3 -> [Vz_Earth_error]
  Demux13/2 -> [Vy_Earth_error]
  Demux13/1 -> [Vx_Earth_error]
  Sum19/1 -> Display6/1, Demux13/1
  Bus Selector/6 -> Earth to EarthPsi/2, Display5/1  "<V_e>"
  Demux14/3 -> [Vz_Earth]
  Demux14/2 -> [Vy_Earth]
  Demux14/1 -> [Vx_Earth]
  Ground3/1 -> Mux12/1
  Ground2/1 -> Mux12/2
  [psi] -> Mux12/3
  Mux12/1 -> Rotation Angles to Direction Cosine Matrix/1
  Rotation Angles to Direction Cosine Matrix/1 -> Earth to EarthPsi/1
  Mux10/1 -> Sum19/2
  Earth to EarthPsi/1 -> Sum19/1, Display7/1, Demux14/1, [V_Earth]
  PID Controller3/1 -> Display8/1, [theta_ref]  "theta_ref"
  PID Controller4/1 -> Display9/1, [phi_ref]  "phi_ref"
  Bus Selector/7 -> [acc_b]  "<A_b>"
  [euler_dot] -> Mux13/2
  [acc_b] -> Selector2/1
  [v_ad] -> Scope/1  "v_ad"
  Mux13/1 -> Sum20/2  "y_dot"
  [v] -> Sum20/1
  Sum20/1 -> Scope/2  "inv_error"
  Selector2/1 -> Trimmed actuator signals8/1, Mux13/1
  Product1/1 -> Trimmed actuator signals9/1
  Selector3/1 -> Product1/2
  Bus Selector/8 -> [acc_s]  "<A_s>"
  [gforce_body] -> Sum21/2
  [acc_b] -> Sum21/1
  Sum21/1 -> Trimmed actuator signals10/1

== system lib_controller/Controller/NDI+CA Controller/4DOF NDI+CA Controller ==
  note: This DCM is Tb->e
      | Xbody = DCM x Xearth
  measurements : Inport
  earth_ref : Inport  Port=2
  trim_control_input : Inport  Port=3
  Bus Selector : BusSelector  OutputSignals=euler,euler_dot,X_e,DCM,V_b
  Demux{,1..8} (9 alike) : Demux  Outputs=3
  Demux9 : Demux  Outputs=9
  Earth to body : Product  Multiplication=Matrix(*)
  F(X) : MATLAB Function  TreatAsAtomicUnit=on
  F(X)1 : MATLAB Function  TreatAsAtomicUnit=on
  Memory : Memory  LinearizeAsDelay=on
  Mux{,1..3} (4 alike) : Mux  Inputs=3
  Sum : Sum  Inputs=|+-
  Sum1 : Sum  Inputs=-+|
  Sum3 : Sum  Inputs=-+|
  Sum4 : Sum  Inputs=|+-
  Controller output : Outport
  wires:
  Mux/1 -> Sum/1
  Demux3/3 -> [r]
  Demux3/2 -> [q]
  Demux3/1 -> [p]
  Demux2/1 -> [phi]
  Demux2/2 -> [theta]
  Demux2/3 -> [psi]
  measurements/1 -> Bus Selector/1
  Bus Selector/1 -> Demux2/1, Sum/2  "<euler>"
  Bus Selector/2 -> Demux3/1, Sum1/1  "<euler_dot>"
  Sum1/1 -> Demux/1
  Sum/1 -> Demux1/1
  Demux/3 -> [r_error]
  Demux/2 -> [q_error]
  Demux/1 -> [p_error]
  Demux1/1 -> [phi_error]
  Demux1/2 -> [theta_error]
  Demux1/3 -> [psi_error]
  trim_control_input/1 -> [trimmed_input]
  [theta_ref] -> Mux/2
  [phi_ref] -> Mux/1
  [psi_ref] -> Mux/3
  Mux2/1 -> Sum1/2
  [q_ref] -> Mux2/2
  [p_ref] -> Mux2/1
  [r_ref] -> Mux2/3
  Bus Selector/3 -> Demux5/1, Sum3/1  "<X_e>"
  Demux5/3 -> [Z_earth]
  Demux5/2 -> [Y_earth]
  Demux5/1 -> [X_earth]
  Demux4/3 -> [z_error]
  Demux4/2 -> [y_error]
  Demux4/1 -> [x_error]
  Mux1/1 -> Sum3/2
  [Yearth_ref] -> Mux1/2
  [Xearth_ref] -> Mux1/1
  [Zearth_ref] -> Mux1/3
  Mux3/1 -> Sum4/1
  Demux7/1 -> [vx_b]
  Demux7/2 -> [vy_b]
  Demux7/3 -> [vz_b]
  Bus Selector/5 -> Demux7/1, Sum4/2  "<V_b>"
  Sum4/1 -> Demux6/1
  Demux6/1 -> [vx_error]
  Demux6/2 -> [vy_error]
  Demux6/3 -> [vz_error]
  [Vy_body_ref] -> Mux3/2
  [Vx_body_ref] -> Mux3/1
  [Vz_body_ref] -> Mux3/3
  Bus Selector/4 -> Earth to body/2  "<DCM>"
  Earth to body/1 -> Demux4/1
  Sum3/1 -> Earth to body/1
  Demux8/3 -> [Zearth_ref]
  Demux8/2 -> [Yearth_ref]
  Demux8/1 -> [Xearth_ref]
  earth_ref/1 -> Demux8/1
  [prev_output] -> Demux9/1
  Demux9/1 -> [throttle1_0]
  Demux9/2 -> [eta1_0]
  Demux9/3 -> [gamma1_0]
  Demux9/4 -> [throttle2_0]
  Demux9/5 -> [eta2_0]
  Demux9/6 -> [gamma2_0]
  Demux9/7 -> [throttle3_0]
  Demux9/8 -> [eta3_0]
  Demux9/9 -> [gamma3_0]
  ? -> Controller output/1, Memory/1
  Memory/1 -> [prev_output]
